simulink library "simulink_lib"  (R2016a)
settings: Solver=ode45  StartTime=0.0  StopTime=10.0  RelTol=1e-3
libraries: simulink_lib x7
settings Model: Creator=Mario  LastModifiedBy=Mario
settings DataIOCC: LimitDataPoints=on
settings DebuggingCC: AllowSymbolicDim=off

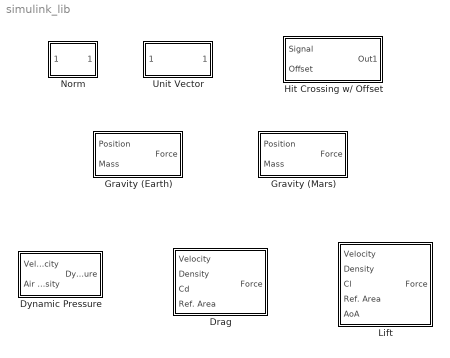
== system simulink_lib ==
  Drag : Subsystem  mask(Drag){}
  Dynamic Pressure : Subsystem  mask(Dynamic Pressure){}
  Gravity (Earth) : Subsystem  mask(Gravity (Earth)){}
      mask help: Calculates gravitational force for Earth.
  Gravity (Mars) : Subsystem  mask(Gravity (Mars)){}
      mask help: Calculates gravitational force for Mars.
  Hit Crossing w/ Offset : Subsystem  mask(Hit Crossing w/ Input){direction=Either}
      mask prompts: direction "Direction for hit crossing detection."
      mask help: Hit crossing block with offset input.
      mask TypeOptions direction: Rising | Falling | Either
      mask DialogControl DescTextVar Prompt: Hit crossing detection with accessible offset.
  Lift : Subsystem  mask(Lift){}
  Norm : Subsystem  mask(Norm){}
      mask help: Calculates the norm of a vector.
      mask Display: disp('Norm')
  Unit Vector : Subsystem  mask(Unit Vector){}
      mask help: Normalizes vector.
      mask Display: disp('Unit Vector')

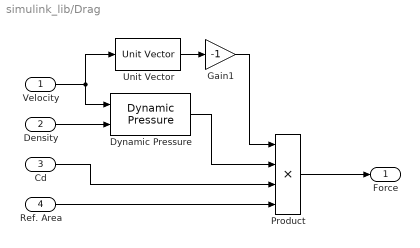
== system simulink_lib/Drag ==
  Velocity : Inport
  Density : Inport  Port=2
  Cd : Inport  Port=3
  Ref. Area : Inport  Port=4
  Dynamic Pressure : simulink_lib/Dynamic Pressure  SystemSampleTime=-1
  Gain1 : Gain  Gain=-1
  Product : Product  Inputs=4
  Unit Vector : simulink_lib/Unit Vector
  Force : Outport
  wires:
  Unit Vector/1 -> Gain1/1
  Velocity/1 -> Dynamic Pressure/1, Unit Vector/1
  Density/1 -> Dynamic Pressure/2
  Dynamic Pressure/1 -> Product/2
  Ref. Area/1 -> Product/4
  Cd/1 -> Product/3
  Gain1/1 -> Product/1
  Product/1 -> Force/1

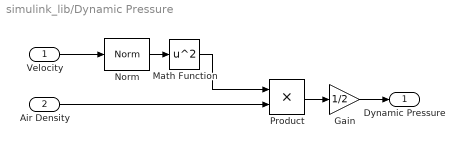
== system simulink_lib/Dynamic Pressure ==
  Velocity : Inport
  Air Density : Inport  Port=2
  Gain : Gain  Gain=1/2
  Math Function : Math  Operator=square  SaturateOnIntegerOverflow=on
  Norm : simulink_lib/Norm
  Product : Product
  Dynamic Pressure : Outport
  wires:
  Velocity/1 -> Norm/1
  Norm/1 -> Math Function/1
  Math Function/1 -> Product/1
  Air Density/1 -> Product/2
  Product/1 -> Gain/1
  Gain/1 -> Dynamic Pressure/1

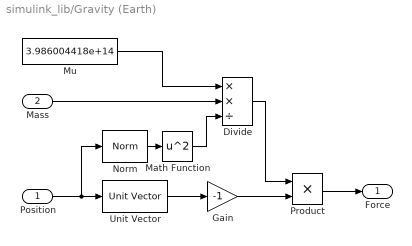
== system simulink_lib/Gravity (Earth) ==
  Position : Inport
  Mass : Inport  Port=2
  Divide : Product  Inputs=**/  RndMeth=Round
  Gain : Gain  Gain=-1
  Math Function : Math  Operator=square  SaturateOnIntegerOverflow=on
  Mu : Constant  Value=3.986004418e+14
  Norm : simulink_lib/Unit Vector/Norm
  Product : Product
  Unit Vector : simulink_lib/Unit Vector
  Force : Outport
  wires:
  Position/1 -> Norm/1, Unit Vector/1
  Unit Vector/1 -> Gain/1
  Mu/1 -> Divide/1
  Mass/1 -> Divide/2
  Gain/1 -> Product/2
  Product/1 -> Force/1
  Divide/1 -> Product/1
  Norm/1 -> Math Function/1
  Math Function/1 -> Divide/3

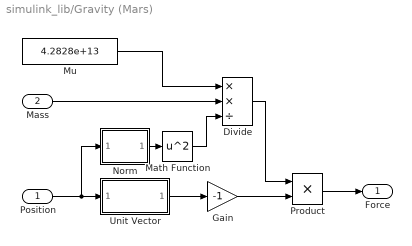
== system simulink_lib/Gravity (Mars) ==
  Position : Inport
  Mass : Inport  Port=2
  Divide : Product  Inputs=**/  RndMeth=Round
  Gain : Gain  Gain=-1
  Math Function : Math  Operator=square  SaturateOnIntegerOverflow=on
  Mu : Constant  Value=4.2828e+13
  Norm : Subsystem  mask(Norm){}
      mask help: Calculates the norm of a vector.
      mask Display: disp('Norm')
  Product : Product
  Unit Vector : Subsystem  mask(Unit Vector){}
      mask help: Normalizes vector.
      mask Display: disp('Unit Vector')
  Force : Outport
  wires:
  Math Function/1 -> Divide/3
  Norm/1(Norm) -> Math Function/1
  Divide/1 -> Product/1
  Product/1 -> Force/1
  Gain/1 -> Product/2
  Mass/1 -> Divide/2
  Mu/1 -> Divide/1
  Unit Vector/1(Unit Vector) -> Gain/1
  Position/1 -> Unit Vector/1(Vector), Norm/1(Vector)

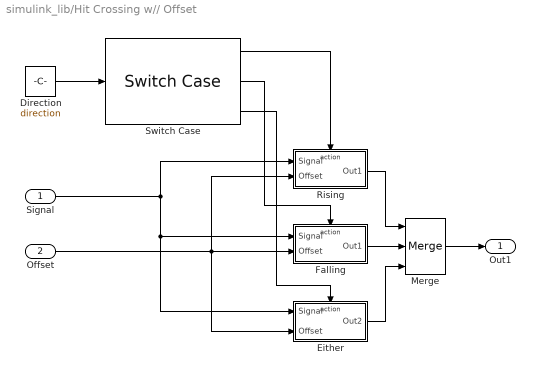
== system simulink_lib/Hit Crossing w// Offset ==
  Signal : Inport
  Offset : Inport  Port=2
  Direction : Constant  Value=direction
  Either : Subsystem  TreatAsAtomicUnit=on
  Falling : Subsystem  TreatAsAtomicUnit=on
  Merge : Merge  Inputs=3
  Rising : Subsystem  TreatAsAtomicUnit=on
  Switch Case : SwitchCase  CaseConditions={1,2,3}  ShowDefaultCase=off
  Out1 : Outport  OutDataTypeStr=boolean
  wires:
  Direction/1 -> Switch Case/1
  Switch Case/2 -> Falling/Action
  Switch Case/1 -> Rising/Action
  Switch Case/3 -> Either/Action
  Falling/1(Out1) -> Merge/2
  Merge/1 -> Out1/1
  Rising/1(Out1) -> Merge/1
  Either/1(Out2) -> Merge/3
  Signal/1 -> Rising/1(Signal), Either/1(Signal), Falling/1(Signal)
  Offset/1 -> Either/2(Offset), Rising/2(Offset), Falling/2(Offset)

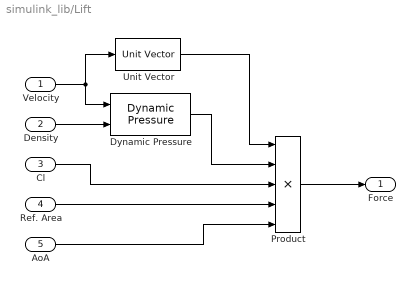
== system simulink_lib/Lift ==
  Velocity : Inport
  Density : Inport  Port=2
  Cl : Inport  Port=3
  Ref. Area : Inport  Port=4
  AoA : Inport  Port=5
  Dynamic Pressure : simulink_lib/Dynamic Pressure  SystemSampleTime=-1
  Product : Product  Inputs=5
  Unit Vector : simulink_lib/Unit Vector
  Force : Outport
  wires:
  Velocity/1 -> Dynamic Pressure/1, Unit Vector/1
  Density/1 -> Dynamic Pressure/2
  Dynamic Pressure/1 -> Product/2
  Ref. Area/1 -> Product/4
  Cl/1 -> Product/3
  Unit Vector/1 -> Product/1
  Product/1 -> Force/1
  AoA/1 -> Product/5

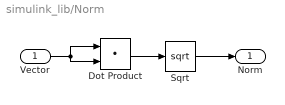
== system simulink_lib/Norm ==
  Vector : Inport
  Dot Product : DotProduct  InputSameDT=on  OutDataTypeStr=Inherit: Inherit via internal rule
  Sqrt : Sqrt  SaturateOnIntegerOverflow=on
  Norm : Outport
  wires:
  Vector/1 -> Dot Product/1, Dot Product/2
  Dot Product/1 -> Sqrt/1
  Sqrt/1 -> Norm/1

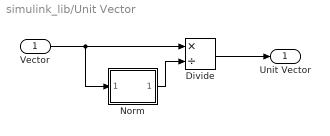
== system simulink_lib/Unit Vector ==
  Vector : Inport
  Divide : Product  Inputs=*/
  Norm : Subsystem  mask(Norm){}
      mask help: Calculates the norm of a vector.
      mask Display: disp('Norm')
  Unit Vector : Outport
  wires:
  Vector/1 -> Divide/1, Norm/1(Vector)
  Norm/1(Norm) -> Divide/2
  Divide/1 -> Unit Vector/1

== system simulink_lib/Gravity (Mars)/Norm ==
  Vector : Inport
  Dot Product : DotProduct  InputSameDT=on  OutDataTypeStr=Inherit: Inherit via internal rule
  Sqrt : Sqrt  SaturateOnIntegerOverflow=on
  Norm : Outport
  wires:
  Sqrt/1 -> Norm/1
  Dot Product/1 -> Sqrt/1
  Vector/1 -> Dot Product/2, Dot Product/1

== system simulink_lib/Gravity (Mars)/Unit Vector ==
  Vector : Inport
  Divide : Product  Inputs=*/
  Norm : Subsystem  mask(Norm){}
      mask help: Calculates the norm of a vector.
      mask Display: disp('Norm')
  Unit Vector : Outport
  wires:
  Divide/1 -> Unit Vector/1
  Norm/1(Norm) -> Divide/2
  Vector/1 -> Norm/1(Vector), Divide/1

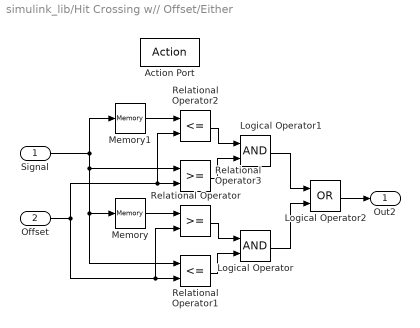
== system simulink_lib/Hit Crossing w// Offset/Either ==
  Signal : Inport
  Offset : Inport  Port=2
  Action Port : ActionPort  InitializeStates=reset
  Logical Operator : Logic  AllPortsSameDT=off  OutDataTypeStr=boolean
  Logical Operator1 : Logic  AllPortsSameDT=off  OutDataTypeStr=boolean
  Logical Operator2 : Logic  Operator=OR  AllPortsSameDT=off  OutDataTypeStr=boolean
  Memory : Memory  InheritSampleTime=on
  Memory1 : Memory  X0=1e+16  InheritSampleTime=on
  Relational Operator : RelationalOperator  OutDataTypeStr=boolean
  Relational Operator1 : RelationalOperator  Operator=<=  OutDataTypeStr=boolean
  Relational Operator2 : RelationalOperator  Operator=<=  OutDataTypeStr=boolean
  Relational Operator3 : RelationalOperator  OutDataTypeStr=boolean
  Out2 : Outport
  wires:
  Memory/1 -> Relational Operator/1
  Relational Operator1/1 -> Logical Operator/2
  Relational Operator/1 -> Logical Operator/1
  Offset/1 -> Relational Operator/2, Relational Operator1/2, Relational Operator2/2, Relational Operator3/2
  Memory1/1 -> Relational Operator2/1
  Relational Operator3/1 -> Logical Operator1/2
  Relational Operator2/1 -> Logical Operator1/1
  Signal/1 -> Memory1/1, Relational Operator1/1, Memory/1, Relational Operator3/1
  Logical Operator2/1 -> Out2/1
  Logical Operator/1 -> Logical Operator2/2
  Logical Operator1/1 -> Logical Operator2/1

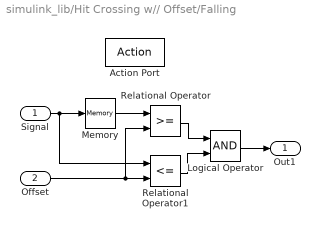
== system simulink_lib/Hit Crossing w// Offset/Falling ==
  Signal : Inport
  Offset : Inport  Port=2
  Action Port : ActionPort  InitializeStates=reset
  Logical Operator : Logic  AllPortsSameDT=off  OutDataTypeStr=boolean
  Memory : Memory  InheritSampleTime=on
  Relational Operator : RelationalOperator  OutDataTypeStr=boolean
  Relational Operator1 : RelationalOperator  Operator=<=  OutDataTypeStr=boolean
  Out1 : Outport
  wires:
  Memory/1 -> Relational Operator/1
  Relational Operator1/1 -> Logical Operator/2
  Relational Operator/1 -> Logical Operator/1
  Signal/1 -> Relational Operator1/1, Memory/1
  Offset/1 -> Relational Operator/2, Relational Operator1/2
  Logical Operator/1 -> Out1/1

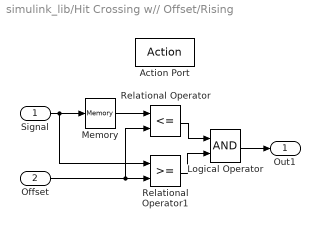
== system simulink_lib/Hit Crossing w// Offset/Rising ==
  Signal : Inport
  Offset : Inport  Port=2
  Action Port : ActionPort  InitializeStates=reset
  Logical Operator : Logic  AllPortsSameDT=off  OutDataTypeStr=boolean
  Memory : Memory  X0=1e+16  InheritSampleTime=on
  Relational Operator : RelationalOperator  Operator=<=  OutDataTypeStr=boolean
  Relational Operator1 : RelationalOperator  OutDataTypeStr=boolean
  Out1 : Outport
  wires:
  Memory/1 -> Relational Operator/1
  Relational Operator1/1 -> Logical Operator/2
  Relational Operator/1 -> Logical Operator/1
  Signal/1 -> Relational Operator1/1, Memory/1
  Offset/1 -> Relational Operator/2, Relational Operator1/2
  Logical Operator/1 -> Out1/1

== system simulink_lib/Unit Vector/Norm ==
  Vector : Inport
  Dot Product : DotProduct  InputSameDT=on  OutDataTypeStr=Inherit: Inherit via internal rule
  Sqrt : Sqrt  SaturateOnIntegerOverflow=on
  Norm : Outport
  wires:
  Vector/1 -> Dot Product/1, Dot Product/2
  Dot Product/1 -> Sqrt/1
  Sqrt/1 -> Norm/1

== system simulink_lib/Gravity (Mars)/Unit Vector/Norm ==
  Vector : Inport
  Dot Product : DotProduct  InputSameDT=on  OutDataTypeStr=Inherit: Inherit via internal rule
  Sqrt : Sqrt  SaturateOnIntegerOverflow=on
  Norm : Outport
  wires:
  Sqrt/1 -> Norm/1
  Dot Product/1 -> Sqrt/1
  Vector/1 -> Dot Product/2, Dot Product/1
